simulink model "cascade_controller"  (R2025a)
settings: Solver=ode4  StartTime=0.0  StopTime=2.0  FixedStep=Ts_plant  RelTol=1e-3
undefined symbols (not defined in the file): enable_notch, Ki_vel, Kp_pos, Kp_vel, tau_max, Ts_pos, Ts_vel
libraries: slpidlib x1
settings Model: Creator=yk  LastModifiedBy=yk

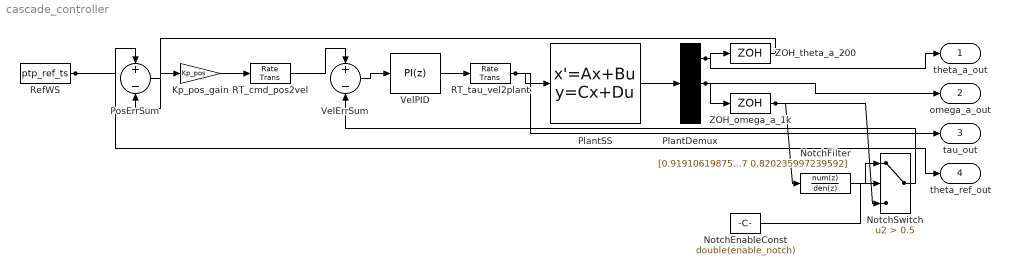
== system cascade_controller ==
  Kp_pos_gain : Gain  Gain=Kp_pos
  NotchEnableConst : Constant  Value=double(enable_notch)
  NotchFilter : DiscreteFilter  Numerator=[0.919106198757816 -1.78799461340587 0.901129798481775]  Denominator=[1 -1.78799461340587 0.820235997239592]  SampleTime=Ts_vel
  NotchSwitch : Switch  Criteria=u2 > Threshold  Threshold=0.5  SaturateOnIntegerOverflow=off  InputSameDT=off
  PlantDemux : Demux  Outputs=3
  PlantSS : StateSpace  A=[0 1 0 0;-29610 -15 29610 5;0 0 0 1;5922 1 -5922 -5]  B=[0;1000;0;0]  C=[0 0 1 0;0 0 0 1;1 0 0 0]  D=[0;0;0]  InitialCondition=0
  PosErrSum : Sum  Inputs=+-
  RT_cmd_pos2vel : RateTransition
  RT_tau_vel2plant : RateTransition
  RefWS : FromWorkspace  VariableName=ptp_ref_ts  SampleTime=Ts_pos
  VelErrSum : Sum  Inputs=+-
  VelPID : slpidlib/PID Controller  Controller=PI  Form=Parallel  TimeDomain=Discrete-time  UseExternalTs=off  SampleTime=Ts_vel  IntegratorMethod=Forward Euler  FilterMethod=Forward Euler  ControllerParametersSource=internal  P=Kp_vel  I=Ki_vel  UseKiTs=off  D=0  UseExternalDerivativeSource=off  N=100  UseFilter=on  TunerSelectOption=Transfer Function Based (PID Tuner App)  InitialConditionSource=internal  InitialConditionForIntegrator=0  InitialConditionForFilter=0  DifferentiatorICPrevScaledInput=0  ExternalReset=none  TrackingMode=off  Kt=1  LimitOutput=on  SatLimitsSource=internal  UpperSaturationLimit=tau_max  LowerSaturationLimit=-tau_max  LinearizeAsGain=on  AntiWindupMode=back-calculation  Kb=1  LimitIntegrator=off  UpperIntegratorSaturationLimit=inf  LowerIntegratorSaturationLimit=-inf  POutMin=[]  POutMax=[]  IOutMin=[]  IOutMax=[]  DOutMin=[]  DOutMax=[]  NOutMin=[]  NOutMax=[]  SumOutMin=[]  SumOutMax=[]  SaturationOutMin=[]  SaturationOutMax=[]  PParamMin=[]  PParamMax=[]  IParamMin=[]  IParamMax=[]  DParamMin=[]  DParamMax=[]  NParamMin=[]  NParamMax=[]  KbParamMin=[]  KbParamMax=[]  KtParamMin=[]  KtParamMax=[]  KbOutMin=[]  KbOutMax=[]  KtOutMin=[]  KtOutMax=[]  IntegratorOutMin=[]  IntegratorOutMax=[]  FilterOutMin=[]  FilterOutMax=[]  SumI1OutMin=[]  SumI1OutMax=[]  SumI2OutMin=[]  SumI2OutMax=[]  SumI3OutMin=[]  SumI3OutMax=[]  SumI4OutMin=[]  SumI4OutMax=[]  SumDOutMin=[]  SumDOutMax=[]  DifferentiatorOutMin=[]  DifferentiatorOutMax=[]  FilterDiffOutCoefMin=[]  FilterDiffOutCoefMax=[]  ReciprocalOutMin=[]  ReciprocalOutMax=[]  SumDenOutMin=[]  SumDenOutMax=[]  SumNumOutMin=[]  SumNumOutMax=[]  DivideOutMin=[]  DivideOutMax=[]  UdiffTsProdOutMin=[]  UdiffTsProdOutMax=[]  NTsProdOutMin=[]  NTsProdOutMax=[]  UintegralTsProdOutMin=[]  UintegralTsProdOutMax=[]  UngainTsProdOutMin=[]  UngainTsProdOutMax=[]  ClampingZeroOutDataTypeStr=Inherit: Inherit via back propagation  ClampingZeroOutMin=[]  ClampingZeroOutMax=[]  FilterDenConstantOutDataTypeStr=Inherit: Inherit via back propagation  FilterDenConstantOutMin=[]  FilterDenConstantOutMax=[]  PCopyOutDataTypeStr=Inherit: Inherit via back propagation  PCopyOutMin=[]  PCopyOutMax=[]  NCopyOutDataTypeStr=Inherit: Inherit via back propagation  NCopyOutMin=[]  NCopyOutMax=[]  IntegratorContinuousStateAttributes=''  IntegratorStateMustResolveToSignalObject=off  IntegratorRTWStateStorageClass=Auto  FilterContinuousStateAttributes=''  FilterStateMustResolveToSignalObject=off  FilterRTWStateStorageClass=Auto  ParallelPVariant=InternalParameters  IdealPVariant=Disabled  IVariant=InternalParameters  DVariant=Disabled  IntegratorVariant=Discrete  SatVariant=Enabled  AWVariant=BackCalculation  PCopyVariant=Disabled  TRVariant=Disabled  FdbkBlocksVariant=Forward  IdealPFdbkVariant=Disabled  SatFdbkVariant=Disabled  DerivativeFilterVariant=Disabled  NVariant=Disabled  NCopyVariant=Disabled_SignalSpec  FilterICVariant=Disabled  IntegratorICVariant=InternalICs  ExternalResetVariant=Disabled  TRSumVariant=Passthrough  SumFdbkVariant=Disabled  SumVariant=Sum_PI  TsampFilterVariant=InternalTs  TsampNgainVariant=Passthrough  TsampIntegralVariant=Disabled_SignalSpec  ExternalSaturationOutDataTypeStr=Inherit: Same as second input  DerivativeSourceVariant=Disabled  PreIntVariant=InternalPreInt
  ZOH_omega_a_1k : ZeroOrderHold  SampleTime=Ts_vel
  ZOH_theta_a_200 : ZeroOrderHold  SampleTime=Ts_pos
  theta_a_out : Outport
  omega_a_out : Outport  Port=2
  tau_out : Outport  Port=3
  theta_ref_out : Outport  Port=4
  wires:
  RefWS/1 -> PosErrSum/1, theta_ref_out/1
  PosErrSum/1 -> Kp_pos_gain/1
  Kp_pos_gain/1 -> RT_cmd_pos2vel/1
  RT_cmd_pos2vel/1 -> VelErrSum/1
  VelErrSum/1 -> VelPID/1
  VelPID/1 -> RT_tau_vel2plant/1
  RT_tau_vel2plant/1 -> PlantSS/1, tau_out/1
  PlantSS/1 -> PlantDemux/1
  PlantDemux/1 -> ZOH_theta_a_200/1, theta_a_out/1
  PlantDemux/2 -> ZOH_omega_a_1k/1, omega_a_out/1
  ZOH_theta_a_200/1 -> PosErrSum/2
  ZOH_omega_a_1k/1 -> NotchFilter/1, NotchSwitch/3
  NotchFilter/1 -> NotchSwitch/1
  NotchEnableConst/1 -> NotchSwitch/2
  NotchSwitch/1 -> VelErrSum/2
